simulink model "c28x_CAN_comm"  (R2021b)
settings: Solver=FixedStepDiscrete  StartTime=0.0  StopTime=Inf  RelTol=1e-3  EnableMultiTasking=on
libraries: c280xlib x2, demo_controls x1
settings Model: ExtModeTrigDuration=8  Creator=The MathWorks, Inc.  LastModifiedBy=The MathWorks, Inc.
settings OptimizationCC: DefaultUnderspecifiedDataType=single  EnhancedBackFolding=on  PassReuseOutputArgsAs=Individual arguments  MaxStackSize=1024  OptimizeBlockOrder=speed  DifferentSizesBufferReuse=on  OptimizationCustomize=off  DenormalBehavior=FlushToZero  EfficientTunableParamExpr=on
settings DebuggingCC: ParameterTunabilityLossMsg=error
settings HardwareCC: ProdBitPerChar=16  ProdBitPerInt=16  ProdBitPerPointer=32  ProdBitPerSizeT=32  ProdBitPerPtrDiffT=32  ProdLargestAtomicInteger=Integer  ProdLargestAtomicFloat=None  ProdWordSize=16  ProdLongLongMode=on  ProdHWDeviceType=Texas Instruments->C2000
settings SFSimCC: MATLABDynamicMemAlloc=off
settings RTWCC: Description=Embedded Coder  SystemTargetFile=ert.tlc  HardwareBoard=TI Piccolo F28069M LaunchPad  TemplateMakefile=ert_default_tmf  Toolchain=Texas Instruments Code Composer Studio (C2000)  BuildConfiguration=Debug
settings CodeAppCC: ForceParamTrailComments=on  IgnoreCustomStorageClasses=off  OperatorAnnotations=on  SimulinkDataObjDesc=on  SFDataObjDesc=on  InsertBlockDesc=on
settings ERTTargetCC: CodeReplacementLibrary=TI C28x  ExtModeTransport=3  ExtModeStaticAlloc=on  ExtModeStaticAllocSize=10000

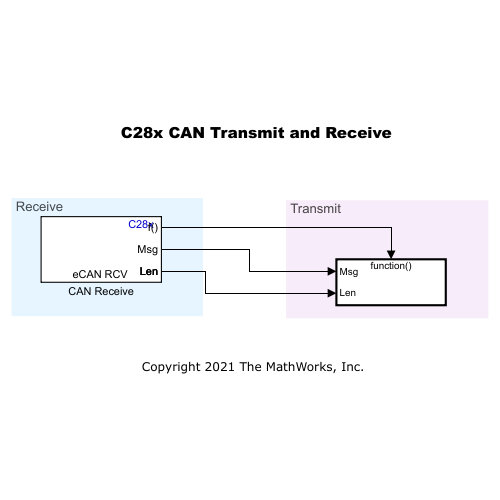
[thumbnail: Simulink's stored preview of the top-level diagram]
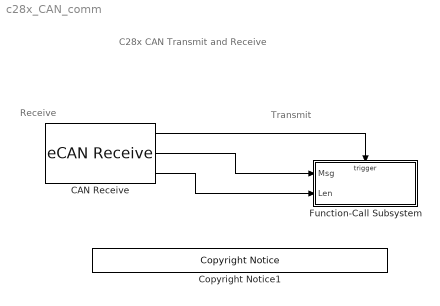
== system c28x_CAN_comm ==
  note: Receive
  note: Transmit
  note: C28x CAN Transmit and Receive
  CAN Receive : c280xlib/eCAN Receive  chipFamily=C280x  useModule=eCAN_A  mailboxNo=2  messageID=hex2dec('0x0000037B')  messageType=Standard (11-bit identifier)  enableAcceptanceFiltering=off  messageIDMask=hex2dec('0x00000007')  sampleTime=0.05  dataType=uint8  outputAction=Output last received values  initValue=255  outputMessageID=on  outputMessageLength=on  outputMessageTimeStamp=off  postInterrupt=off  interruptLine=0
      settings: SourceProductBaseCode=TIC2000
  Copyright Notice1 : demo_controls/Copyright Notice  year=2021  prod=tic2000
      settings: SourceProductBaseCode=ME
  Function-Call Subsystem : Subsystem  TreatAsAtomicUnit=on
  wires:
  CAN Receive/1 -> Function-Call Subsystem/Trigger
  CAN Receive/2 -> Function-Call Subsystem/1(Msg)
  CAN Receive/3 -> Function-Call Subsystem/2(Len)

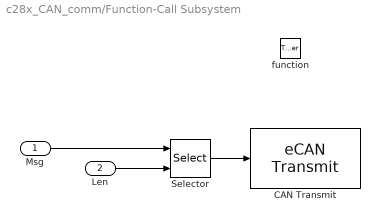
== system c28x_CAN_comm/Function-Call Subsystem ==
  Msg : Inport
  Len : Inport  Port=2
  function : TriggerPort  TriggerType=function-call  VariantControl=(inherit)
  CAN Transmit : c280xlib/eCAN Transmit  chipFamily=C280x  useModule=eCAN_A  mailboxNo=1  messageID=hex2dec('0x0000000C')  messageType=Standard (11-bit identifier)  enableBlockingMode=off  postInterrupt=off  interruptLine=0
      settings: SourceProductBaseCode=TIC2000
  Selector : Selector  InputPortWidth=8  IndexOptions=Starting index (port)  Indices=[1 3]  OutputSizes=1
  wires:
  Msg/1 -> Selector/1
  Len/1 -> Selector/2
  Selector/1 -> CAN Transmit/1
